simulink model "UnRealDataPackaging"  (R2020a)
settings: Solver=FixedStepDiscrete  StartTime=0.0  StopTime=inf  FixedStep=0.02  RelTol=1e-3
libraries: etargetslib x2, dspnetwork x1
settings Model: Creator=kcx06  LastModifiedBy=kcx06
settings SolverCC: AutoInsertRateTranBlk=on
settings DataIOCC: SaveOutput=off  SignalLogging=off  DSMLogging=off  SaveTime=off
settings DebuggingCC: RootOutportRequireBusObject=error  StrictBusMsg=ErrorOnBusTreatedAsVector  ArithmeticOperatorsInVariantConditions=warning
settings ModelReferenceCC: ModelReferenceNumInstancesAllowed=Single
settings SFSimCC: SimUseLocalCustomCode=off  CustomCodeUndefinedFunction=UseInterfaceOnly
settings RTWCC: Description=Generic Real-Time Target  RTWUseLocalCustomCode=off
settings CodeAppCC: StateflowObjectComments=on

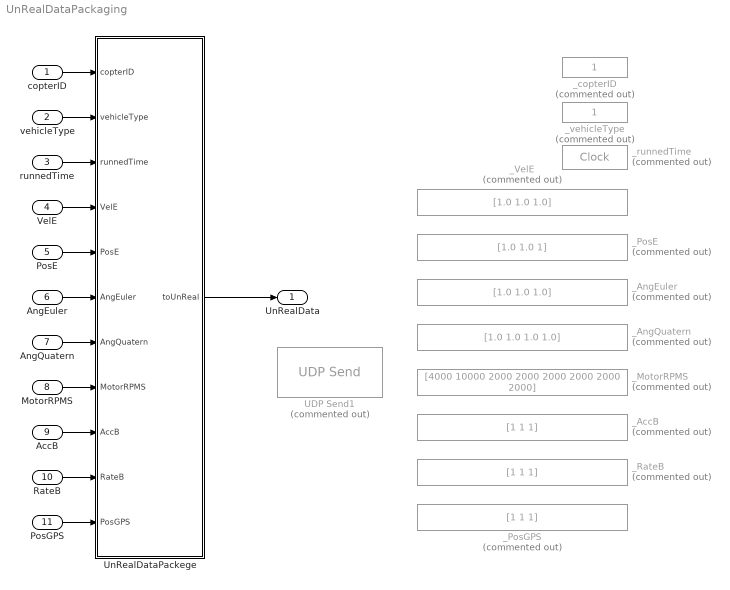
== system UnRealDataPackaging ==
  copterID : Inport  PortDimensions=1
  vehicleType : Inport  Port=2  PortDimensions=1
  runnedTime : Inport  Port=3  PortDimensions=1
  VelE : Inport  Port=4  PortDimensions=3
  PosE : Inport  Port=5  PortDimensions=3
  AngEuler : Inport  Port=6  PortDimensions=3
  AngQuatern : Inport  Port=7  PortDimensions=4
  MotorRPMS : Inport  Port=8  PortDimensions=8
  AccB : Inport  Port=9  PortDimensions=3
  RateB : Inport  Port=10  PortDimensions=3
  PosGPS : Inport  Port=11  PortDimensions=3
  UDP Send1 : dspnetwork/UDP Send  Commented=on  remoteURL='255.255.255.255'  remotePort=20010  localURL='0.0.0.0'  localPortSource=Automatically determine  localPort=20011  sendBufferSize=8192  sampletime=-1  blockPlatform=[]  separateLengthPort=0
  UnRealDataPackege : Subsystem  TreatAsAtomicUnit=on
  _AccB : Constant  Commented=on  Value=[1 1 1]  OutDataTypeStr=single
  _AngEuler : Constant  Commented=on  Value=[1.0 1.0 1.0]  OutDataTypeStr=single
  _AngQuatern : Constant  Commented=on  Value=[1.0 1.0 1.0 1.0]  OutDataTypeStr=single
  _MotorRPMS : Constant  Commented=on  Value=[4000 10000 2000 2000 2000 2000 2000 2000]  OutDataTypeStr=single
  _PosE : Constant  Commented=on  Value=[1.0 1.0 1]  OutDataTypeStr=single
  _PosGPS : Constant  Commented=on  Value=[1 1 1]  OutDataTypeStr=double
  _RateB : Constant  Commented=on  Value=[1 1 1]  OutDataTypeStr=single
  _VelE : Constant  Commented=on  Value=[1.0 1.0 1.0]  OutDataTypeStr=single
  _copterID : Constant  Commented=on  OutDataTypeStr=Inherit: Inherit via back propagation
  _runnedTime : DigitalClock  Commented=on  SampleTime=0.01
  _vehicleType : Constant  Commented=on  OutDataTypeStr=Inherit: Inherit via back propagation
  UnRealData : Outport
  wires:
  UnRealDataPackege/1(toUnReal) -> UnRealData/1
  PosGPS/1 -> UnRealDataPackege/11(PosGPS)
  RateB/1 -> UnRealDataPackege/10(RateB)
  AccB/1 -> UnRealDataPackege/9(AccB)
  MotorRPMS/1 -> UnRealDataPackege/8(MotorRPMS)
  AngQuatern/1 -> UnRealDataPackege/7(AngQuatern)
  AngEuler/1 -> UnRealDataPackege/6(AngEuler)
  PosE/1 -> UnRealDataPackege/5(PosE)
  VelE/1 -> UnRealDataPackege/4("VelE ")
  runnedTime/1 -> UnRealDataPackege/3(runnedTime)
  vehicleType/1 -> UnRealDataPackege/2(vehicleType)
  copterID/1 -> UnRealDataPackege/1(copterID)

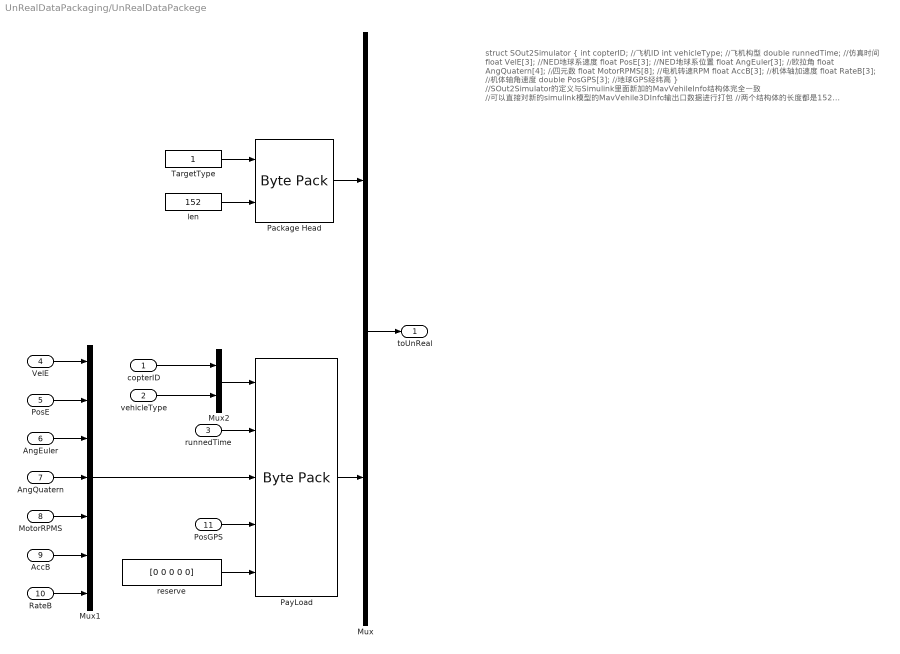
== system UnRealDataPackaging/UnRealDataPackege ==
  note: struct SOut2Simulator
      | {
      | int copterID; //飞机ID
      | int vehicleType; //飞机构型
      | double runnedTime; //仿真时间
      | float VelE[3]; //NED地球系速度
      | float PosE[3]; //NED地球系位置
      | float AngEuler[3]; //欧拉角
      | float AngQuatern[4]; //四元数
      | float MotorRPMS[8]; //电机转速RPM
      | float AccB[3]; //机体轴加速度
      | float RateB[3]; //机体轴角速度
      | double PosGPS[3]; //地球GPS经纬高
      | }
      |
      | //SOut2Simulator的定义与Simulink里面新加的MavVehileInfo结构体完全一致
      | //可以直接对新的simulink模型的MavVehile3DInfo输出口数据进行打包
      | //两个结构体的长度都是152
      | sizeof(SOut2Simulator) = sizeof(MavVehileInfo) = 152
      |
      | 打包封装的结构体为
      | typedef struct _netDataShort
      | {
      | TargetType tg; //这里目前随便填，写1即可 uint32
      | int len; //这个长度为传输结构体长度，目前是152
      | char payload[192]; //这里面前152位存放了SOut2Simulator结构体数据，后面的40位保留
      | }netDataShort;
      |
      | //UDP包的总长度为200
      | sizeof(netDataShort) = 200
      |
      | //发送的UDP端口号为：20010
  copterID : Inport  PortDimensions=1
  vehicleType : Inport  Port=2  PortDimensions=1
  runnedTime : Inport  Port=3  PortDimensions=1
  "VelE " : Inport  Port=4  PortDimensions=3
  PosE : Inport  Port=5  PortDimensions=3
  AngEuler : Inport  Port=6  PortDimensions=3
  AngQuatern : Inport  Port=7  PortDimensions=4
  MotorRPMS : Inport  Port=8  PortDimensions=8
  AccB : Inport  Port=9  PortDimensions=3
  RateB : Inport  Port=10  PortDimensions=3
  PosGPS : Inport  Port=11  PortDimensions=3
  Mux : Mux  Inputs=2
  Mux1 : Mux  Inputs=7
  Mux2 : Mux  Inputs=2
  Package Head : etargetslib/Byte Pack  datatypes={'uint32','int32'}  byteAlign=4
  PayLoad : etargetslib/Byte Pack  datatypes={'int32','double','single','double','double'}  byteAlign=8
  TargetType : Constant  OutDataTypeStr=Inherit: Inherit via back propagation
  len : Constant  Value=152  OutDataTypeStr=Inherit: Inherit via back propagation
  reserve : Constant  Value=[0 0 0 0 0]  OutDataTypeStr=double  SampleTime=-1
  toUnReal : Outport
  wires:
  Package Head/1 -> Mux/1
  "VelE "/1 -> Mux1/1
  PosE/1 -> Mux1/2
  AngEuler/1 -> Mux1/3
  RateB/1 -> Mux1/7
  AccB/1 -> Mux1/6
  PayLoad/1 -> Mux/2
  Mux/1 -> toUnReal/1
  len/1 -> Package Head/2
  MotorRPMS/1 -> Mux1/5
  TargetType/1 -> Package Head/1
  AngQuatern/1 -> Mux1/4
  runnedTime/1 -> PayLoad/2
  PosGPS/1 -> PayLoad/4
  Mux1/1 -> PayLoad/3
  copterID/1 -> Mux2/1
  vehicleType/1 -> Mux2/2
  Mux2/1 -> PayLoad/1
  reserve/1 -> PayLoad/5
